simulink model "chaotic_controller_gt"  (R2025b)
settings: Solver=FixedStepDiscrete  StartTime=0.0  StopTime=300.0  FixedStep=0.1  RelTol=1e-3
settings Model: Creator=soumya2049  LastModifiedBy=aniket

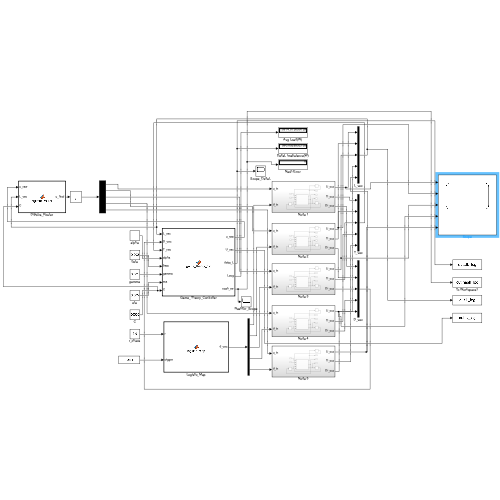
[thumbnail: Simulink's stored preview of the top-level diagram]
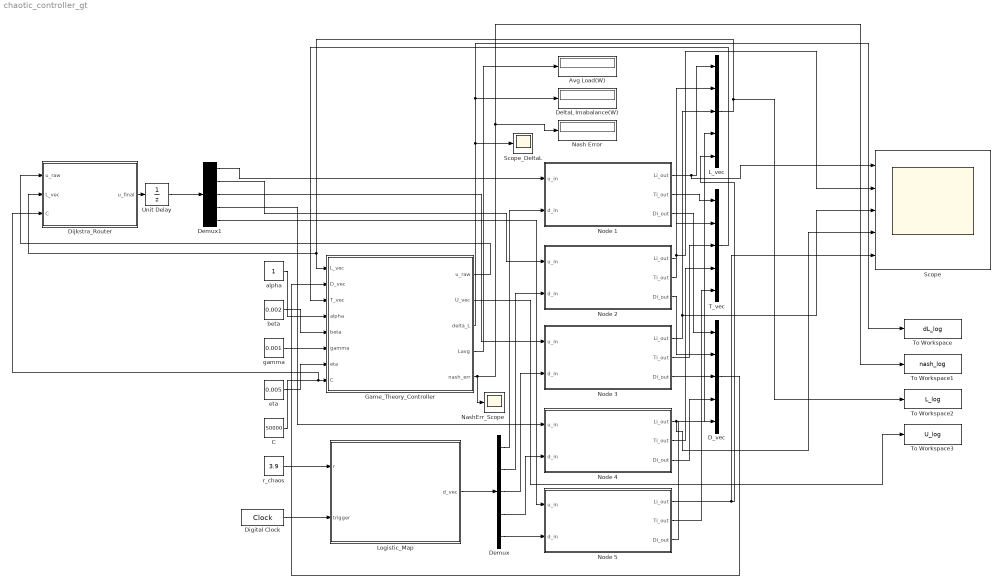
== system chaotic_controller_gt ==
  Avg Load(W) : Display
  C : Constant  Value=50000
  D_vec : Mux  Inputs=5
  DeltaL Imabalance(W) : Display
  Demux : Demux  Outputs=5
  Demux1 : Demux  Outputs=5
  Digital Clock : DigitalClock
  Dijkstra_Router : MATLAB Function  TreatAsAtomicUnit=on
  Game_Theory_Controller : MATLAB Function  TreatAsAtomicUnit=on
  L_vec : Mux  Inputs=5
  Logistic_Map : MATLAB Function  TreatAsAtomicUnit=on
  Nash Error : Display
  NashErr_Scope : Scope
  Node 1 : Subsystem
  Node 2 : Subsystem
  Node 3 : Subsystem
  Node 4 : Subsystem
  Node 5 : Subsystem
  Scope : Scope  NumInputPorts=5
      settings: ActiveDisplayYMinimum=-1436.8341921945957  ActiveDisplayYMaximum=13231.507729751364  DataLoggingVariableName=ScopeData2
  Scope_DeltaL : Scope
      settings: ActiveDisplayYMinimum=-1  ActiveDisplayYMaximum=1
  T_vec : Mux  Inputs=5
  To Workspace : ToWorkspace  VariableName=dL_log  SampleTime=-1
  To Workspace1 : ToWorkspace  VariableName=nash_log  SampleTime=-1
  To Workspace2 : ToWorkspace  VariableName=L_log  SampleTime=-1
  To Workspace3 : ToWorkspace  VariableName=U_log  SampleTime=-1
  Unit Delay : UnitDelay  InitialCondition=zeros(5,1)  SampleTime=-1  HasFrameUpgradeWarning=on
  alpha : Constant
  beta : Constant  Value=0.002
  eta : Constant  Value=0.005
  gamma : Constant  Value=0.001
  r_chaos : Constant  Value=3.9
  wires:
  Digital Clock/1 -> Logistic_Map/2(trigger)
  alpha/1 -> Game_Theory_Controller/4(alpha)
  Node 2/2(Ti_out) -> Scope/2, T_vec/2
  C/1 -> Dijkstra_Router/3(C), Game_Theory_Controller/8(C)
  beta/1 -> Game_Theory_Controller/5(beta)
  gamma/1 -> Game_Theory_Controller/6(gamma)
  r_chaos/1 -> Logistic_Map/1(r)
  Node 3/3(Di_out) -> D_vec/3
  eta/1 -> Game_Theory_Controller/7(eta)
  Logistic_Map/1(d_vec) -> Demux/1
  Demux/1 -> Node 1/2(d_in)
  Node 5/1(Li_out) -> Scope/5, L_vec/5
  Demux/2 -> Node 2/2(d_in)
  Demux/3 -> Node 3/2(d_in)
  Demux/4 -> Node 4/2(d_in)
  Demux/5 -> Node 5/2(d_in)
  Node 1/1(Li_out) -> Scope/1, L_vec/1
  Node 1/2(Ti_out) -> T_vec/1
  Node 5/3(Di_out) -> D_vec/5
  Node 1/3(Di_out) -> D_vec/1
  Node 2/1(Li_out) -> L_vec/2
  Node 2/3(Di_out) -> D_vec/2
  Node 3/1(Li_out) -> Scope/3, L_vec/3
  Node 3/2(Ti_out) -> T_vec/3
  Node 4/1(Li_out) -> Scope/4, L_vec/4
  Node 4/2(Ti_out) -> T_vec/4
  Node 4/3(Di_out) -> D_vec/4
  Node 5/2(Ti_out) -> T_vec/5
  L_vec/1 -> To Workspace2/1, Game_Theory_Controller/1(L_vec), Dijkstra_Router/2(L_vec)
  T_vec/1 -> Game_Theory_Controller/3(T_vec)
  D_vec/1 -> Game_Theory_Controller/2(D_vec)
  Game_Theory_Controller/1(u_raw) -> Dijkstra_Router/1(u_raw)
  Demux1/2 -> Node 2/1(u_in)
  Demux1/3 -> Node 3/1(u_in)
  Demux1/4 -> Node 4/1(u_in)
  Demux1/5 -> Node 5/1(u_in)
  Dijkstra_Router/1(u_final) -> Unit Delay/1
  Unit Delay/1 -> Demux1/1
  Game_Theory_Controller/3(delta_L) -> DeltaL Imabalance(W)/1, To Workspace/1, Scope_DeltaL/1
  Game_Theory_Controller/5(nash_err) -> Nash Error/1, To Workspace1/1, NashErr_Scope/1
  Game_Theory_Controller/2(U_vec) -> To Workspace3/1
  Game_Theory_Controller/4(Lavg) -> Avg Load(W)/1
  Demux1/1 -> Node 1/1(u_in)

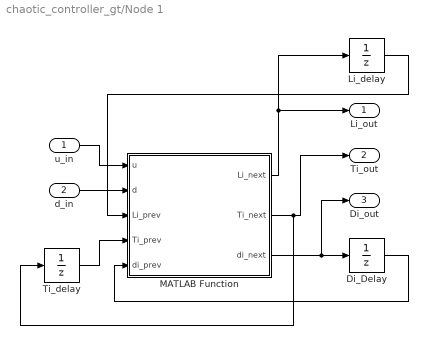
== system chaotic_controller_gt/Node 1 ==
  u_in : Inport
  d_in : Inport  Port=2
  Di_Delay : UnitDelay  InitialCondition=5000  SampleTime=-1  HasFrameUpgradeWarning=on
  Li_delay : UnitDelay  InitialCondition=3000  SampleTime=-1  HasFrameUpgradeWarning=on
  MATLAB Function : MATLAB Function  TreatAsAtomicUnit=on
  Ti_delay : UnitDelay  InitialCondition=30  SampleTime=-1  HasFrameUpgradeWarning=on
  Li_out : Outport
  Ti_out : Outport  Port=2
  Di_out : Outport  Port=3
  wires:
  MATLAB Function/2(Ti_next) -> Ti_delay/1, Ti_out/1
  u_in/1 -> MATLAB Function/1(u)
  d_in/1 -> MATLAB Function/2(d)
  Ti_delay/1 -> MATLAB Function/4(Ti_prev)
  MATLAB Function/1(Li_next) -> Li_out/1, Li_delay/1
  Di_Delay/1 -> MATLAB Function/5(di_prev)
  MATLAB Function/3(di_next) -> Di_out/1, Di_Delay/1
  Li_delay/1 -> MATLAB Function/3(Li_prev)

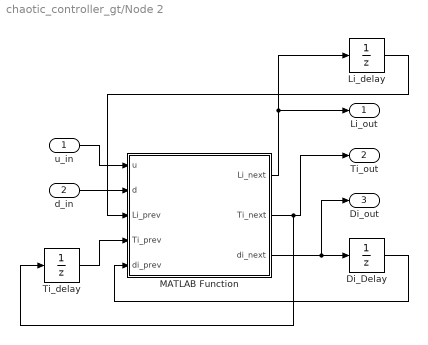
== system chaotic_controller_gt/Node 2 ==
  u_in : Inport
  d_in : Inport  Port=2
  Di_Delay : UnitDelay  InitialCondition=5000  SampleTime=-1  HasFrameUpgradeWarning=on
  Li_delay : UnitDelay  InitialCondition=3000  SampleTime=-1  HasFrameUpgradeWarning=on
  MATLAB Function : MATLAB Function  TreatAsAtomicUnit=on
  Ti_delay : UnitDelay  InitialCondition=30  SampleTime=-1  HasFrameUpgradeWarning=on
  Li_out : Outport
  Ti_out : Outport  Port=2
  Di_out : Outport  Port=3
  wires:
  MATLAB Function/2(Ti_next) -> Ti_delay/1, Ti_out/1
  u_in/1 -> MATLAB Function/1(u)
  d_in/1 -> MATLAB Function/2(d)
  Ti_delay/1 -> MATLAB Function/4(Ti_prev)
  MATLAB Function/1(Li_next) -> Li_out/1, Li_delay/1
  Di_Delay/1 -> MATLAB Function/5(di_prev)
  MATLAB Function/3(di_next) -> Di_out/1, Di_Delay/1
  Li_delay/1 -> MATLAB Function/3(Li_prev)

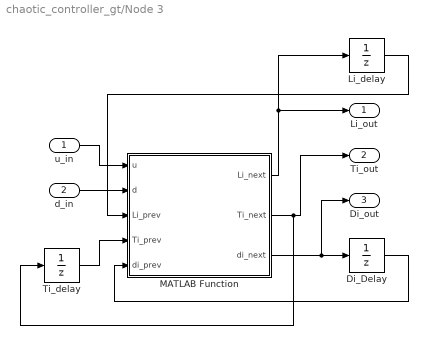
== system chaotic_controller_gt/Node 3 ==
  u_in : Inport
  d_in : Inport  Port=2
  Di_Delay : UnitDelay  InitialCondition=5000  SampleTime=-1  HasFrameUpgradeWarning=on
  Li_delay : UnitDelay  InitialCondition=3000  SampleTime=-1  HasFrameUpgradeWarning=on
  MATLAB Function : MATLAB Function  TreatAsAtomicUnit=on
  Ti_delay : UnitDelay  InitialCondition=30  SampleTime=-1  HasFrameUpgradeWarning=on
  Li_out : Outport
  Ti_out : Outport  Port=2
  Di_out : Outport  Port=3
  wires:
  MATLAB Function/2(Ti_next) -> Ti_delay/1, Ti_out/1
  u_in/1 -> MATLAB Function/1(u)
  d_in/1 -> MATLAB Function/2(d)
  Ti_delay/1 -> MATLAB Function/4(Ti_prev)
  MATLAB Function/1(Li_next) -> Li_out/1, Li_delay/1
  Di_Delay/1 -> MATLAB Function/5(di_prev)
  MATLAB Function/3(di_next) -> Di_out/1, Di_Delay/1
  Li_delay/1 -> MATLAB Function/3(Li_prev)

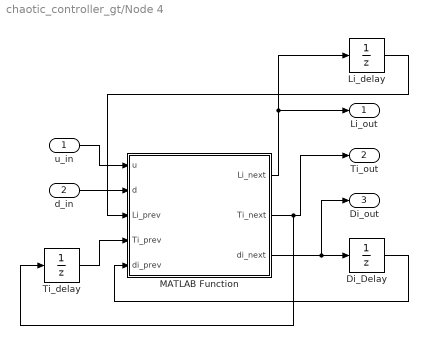
== system chaotic_controller_gt/Node 4 ==
  u_in : Inport
  d_in : Inport  Port=2
  Di_Delay : UnitDelay  InitialCondition=5000  SampleTime=-1  HasFrameUpgradeWarning=on
  Li_delay : UnitDelay  InitialCondition=3000  SampleTime=-1  HasFrameUpgradeWarning=on
  MATLAB Function : MATLAB Function  TreatAsAtomicUnit=on
  Ti_delay : UnitDelay  InitialCondition=30  SampleTime=-1  HasFrameUpgradeWarning=on
  Li_out : Outport
  Ti_out : Outport  Port=2
  Di_out : Outport  Port=3
  wires:
  MATLAB Function/2(Ti_next) -> Ti_delay/1, Ti_out/1
  u_in/1 -> MATLAB Function/1(u)
  d_in/1 -> MATLAB Function/2(d)
  Ti_delay/1 -> MATLAB Function/4(Ti_prev)
  MATLAB Function/1(Li_next) -> Li_out/1, Li_delay/1
  Di_Delay/1 -> MATLAB Function/5(di_prev)
  MATLAB Function/3(di_next) -> Di_out/1, Di_Delay/1
  Li_delay/1 -> MATLAB Function/3(Li_prev)

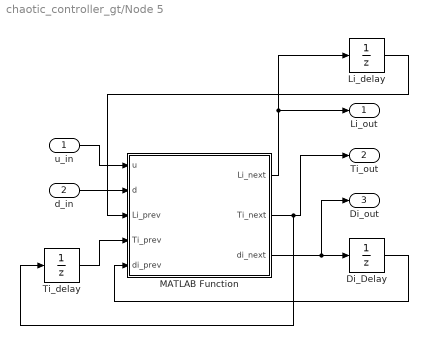
== system chaotic_controller_gt/Node 5 ==
  u_in : Inport
  d_in : Inport  Port=2
  Di_Delay : UnitDelay  InitialCondition=5000  SampleTime=-1  HasFrameUpgradeWarning=on
  Li_delay : UnitDelay  InitialCondition=3000  SampleTime=-1  HasFrameUpgradeWarning=on
  MATLAB Function : MATLAB Function  TreatAsAtomicUnit=on
  Ti_delay : UnitDelay  InitialCondition=30  SampleTime=-1  HasFrameUpgradeWarning=on
  Li_out : Outport
  Ti_out : Outport  Port=2
  Di_out : Outport  Port=3
  wires:
  MATLAB Function/2(Ti_next) -> Ti_delay/1, Ti_out/1
  u_in/1 -> MATLAB Function/1(u)
  d_in/1 -> MATLAB Function/2(d)
  Ti_delay/1 -> MATLAB Function/4(Ti_prev)
  MATLAB Function/1(Li_next) -> Li_out/1, Li_delay/1
  Di_Delay/1 -> MATLAB Function/5(di_prev)
  MATLAB Function/3(di_next) -> Di_out/1, Di_Delay/1
  Li_delay/1 -> MATLAB Function/3(Li_prev)

== matlab function chaotic_controller_gt/Dijkstra_Router ==
  data: u_raw input; u_final output; L_vec input; C input
function u_final = dijkstra_router(u_raw, L_vec, C)
%  u_raw  = 5×1 allocations from game theory (W)
%  L_vec  = 5×1 current loads (W) — used as edge weights
%  C      = capacity limit (W)
%  u_final = 5×1 optimally routed allocations (W)
%
%  DIJKSTRA INTERPRETATION:
%  Nodes = charging stations. Edge weight = current load.
%  "Shortest path" = lowest-load path for power delivery.
%  Heavily loaded nodes get throttled; underloaded get boosted.

total = sum(u_raw);

if total <= C
    u_final = u_raw;   % no congestion — pass through unchanged
    return;
end

%── Model 5 nodes as a weighted graph ─────────────────────────
%  Build a simple adjacency: nodes connected to a central bus
%  Edge weight = current load (W) — high load = costly path
Lavg      = mean(L_vec);
weights   = L_vec / max(L_vec);          % normalise (0 to 1)
distances = weights;                     % Dijkstra "distance" = load weight

%── Sort by Dijkstra distance (lowest load = shortest path) ───
[~, path_order] = sort(distances, 'ascend');  % underloaded nodes get priority

%── Distribute capacity along the optimal path ────────────────
scale   = C / total;
u_final = u_raw * scale;                    % base scaling

%── Redistribute along optimal path: boost underloaded nodes ──
saved = 0;
for k = 5:-1:3                               % top 3 highest-load nodes
    idx           = path_order(k);
    cut           = u_final(idx) * 0.15;      % take 15% from overloaded
    u_final(idx) = u_final(idx) - cut;
    saved         = saved + cut;
end
for k = 1:2                                  % give saved power to 2 underloaded
    idx           = path_order(k);
    u_final(idx) = u_final(idx) + saved/2;
end

%── Safety clamp ──────────────────────────────────────────────
u_final = max(0, min(u_final, 15000));
end

== matlab function chaotic_controller_gt/Node 2/MATLAB Function ==
  data: u input double; Li_next output double; d input double; Li_prev input double; Ti_prev input double; di_prev input double; Ti_next output double; di_next output double
function [Li_next, Ti_next, di_next] = node_dynamics(u, d, Li_prev, Ti_prev, di_prev)
%  u       = allocated power (W) — comes from Dijkstra router
%  d       = chaos disturbance (0 to 1) — from logistic map
%  Li_prev = load at previous timestep (W)
%  Ti_prev = temperature at previous timestep (°C)
%  di_prev = this node's strategy/demand at previous timestep (W)

%  Physical constants
dt    = 0.1;    % sample time (s)
beta  = 0.85;  % charging efficiency (fraction)
alpha = 0.04;  % thermal rise rate (°C per W·s)
eta_t = 0.002; % thermal dissipation coefficient
T_amb = 30;    % ambient temperature (°C)

%  Load update: current draws from allocation, disturbance adds noise
Li_next = Li_prev + dt * (u - beta * Li_prev) + d * 800;

%  Temperature update: rises with power, dissipates toward ambient
Ti_next = Ti_prev + dt * (alpha * u - eta_t * (Ti_prev - T_amb));

%  Strategy: node updates its demand toward allocated value
di_next = di_prev * 0.9 + u * 0.1;  % smoothed demand tracking

%  Hard physical limits
Li_next = max(0, min(Li_next, 15000));   % 0–15 kW
Ti_next = max(20, min(Ti_next, 65));     % 20–65°C
di_next = max(0, min(di_next, 15000));   % 0–15 kW
end

== matlab function chaotic_controller_gt/Node 1/MATLAB Function ==
  data: u input double; Li_next output double; d input double; Li_prev input double; Ti_prev input double; di_prev input double; Ti_next output double; di_next output double
function [Li_next, Ti_next, di_next] = node_dynamics(u, d, Li_prev, Ti_prev, di_prev)
%  u       = allocated power (W) — comes from Dijkstra router
%  d       = chaos disturbance (0 to 1) — from logistic map
%  Li_prev = load at previous timestep (W)
%  Ti_prev = temperature at previous timestep (°C)
%  di_prev = this node's strategy/demand at previous timestep (W)

%  Physical constants
dt    = 0.1;    % sample time (s)
beta  = 0.85;  % charging efficiency (fraction)
alpha = 0.04;  % thermal rise rate (°C per W·s)
eta_t = 0.002; % thermal dissipation coefficient
T_amb = 30;    % ambient temperature (°C)

%  Load update: current draws from allocation, disturbance adds noise
Li_next = Li_prev + dt * (u - beta * Li_prev) + d * 800;

%  Temperature update: rises with power, dissipates toward ambient
Ti_next = Ti_prev + dt * (alpha * u - eta_t * (Ti_prev - T_amb));

%  Strategy: node updates its demand toward allocated value
di_next = di_prev * 0.9 + u * 0.1;  % smoothed demand tracking

%  Hard physical limits
Li_next = max(0, min(Li_next, 15000));   % 0–15 kW
Ti_next = max(20, min(Ti_next, 65));     % 20–65°C
di_next = max(0, min(di_next, 15000));   % 0–15 kW
end

== matlab function chaotic_controller_gt/Node 3/MATLAB Function ==
  data: u input double; Li_next output double; d input double; Li_prev input double; Ti_prev input double; di_prev input double; Ti_next output double; di_next output double
function [Li_next, Ti_next, di_next] = node_dynamics(u, d, Li_prev, Ti_prev, di_prev)
%  u       = allocated power (W) — comes from Dijkstra router
%  d       = chaos disturbance (0 to 1) — from logistic map
%  Li_prev = load at previous timestep (W)
%  Ti_prev = temperature at previous timestep (°C)
%  di_prev = this node's strategy/demand at previous timestep (W)

%  Physical constants
dt    = 0.1;    % sample time (s)
beta  = 0.85;  % charging efficiency (fraction)
alpha = 0.04;  % thermal rise rate (°C per W·s)
eta_t = 0.002; % thermal dissipation coefficient
T_amb = 30;    % ambient temperature (°C)

%  Load update: current draws from allocation, disturbance adds noise
Li_next = Li_prev + dt * (u - beta * Li_prev) + d * 800;

%  Temperature update: rises with power, dissipates toward ambient
Ti_next = Ti_prev + dt * (alpha * u - eta_t * (Ti_prev - T_amb));

%  Strategy: node updates its demand toward allocated value
di_next = di_prev * 0.9 + u * 0.1;  % smoothed demand tracking

%  Hard physical limits
Li_next = max(0, min(Li_next, 15000));   % 0–15 kW
Ti_next = max(20, min(Ti_next, 65));     % 20–65°C
di_next = max(0, min(di_next, 15000));   % 0–15 kW
end

== matlab function chaotic_controller_gt/Node 4/MATLAB Function ==
  data: u input double; Li_next output double; d input double; Li_prev input double; Ti_prev input double; di_prev input double; Ti_next output double; di_next output double
function [Li_next, Ti_next, di_next] = node_dynamics(u, d, Li_prev, Ti_prev, di_prev)
%  u       = allocated power (W) — comes from Dijkstra router
%  d       = chaos disturbance (0 to 1) — from logistic map
%  Li_prev = load at previous timestep (W)
%  Ti_prev = temperature at previous timestep (°C)
%  di_prev = this node's strategy/demand at previous timestep (W)

%  Physical constants
dt    = 0.1;    % sample time (s)
beta  = 0.85;  % charging efficiency (fraction)
alpha = 0.04;  % thermal rise rate (°C per W·s)
eta_t = 0.002; % thermal dissipation coefficient
T_amb = 30;    % ambient temperature (°C)

%  Load update: current draws from allocation, disturbance adds noise
Li_next = Li_prev + dt * (u - beta * Li_prev) + d * 800;

%  Temperature update: rises with power, dissipates toward ambient
Ti_next = Ti_prev + dt * (alpha * u - eta_t * (Ti_prev - T_amb));

%  Strategy: node updates its demand toward allocated value
di_next = di_prev * 0.9 + u * 0.1;  % smoothed demand tracking

%  Hard physical limits
Li_next = max(0, min(Li_next, 15000));   % 0–15 kW
Ti_next = max(20, min(Ti_next, 65));     % 20–65°C
di_next = max(0, min(di_next, 15000));   % 0–15 kW
end

== matlab function chaotic_controller_gt/Node 5/MATLAB Function ==
  data: u input double; Li_next output double; d input double; Li_prev input double; Ti_prev input double; di_prev input double; Ti_next output double; di_next output double
function [Li_next, Ti_next, di_next] = node_dynamics(u, d, Li_prev, Ti_prev, di_prev)
%  u       = allocated power (W) — comes from Dijkstra router
%  d       = chaos disturbance (0 to 1) — from logistic map
%  Li_prev = load at previous timestep (W)
%  Ti_prev = temperature at previous timestep (°C)
%  di_prev = this node's strategy/demand at previous timestep (W)

%  Physical constants
dt    = 0.1;    % sample time (s)
beta  = 0.85;  % charging efficiency (fraction)
alpha = 0.04;  % thermal rise rate (°C per W·s)
eta_t = 0.002; % thermal dissipation coefficient
T_amb = 30;    % ambient temperature (°C)

%  Load update: current draws from allocation, disturbance adds noise
Li_next = Li_prev + dt * (u - beta * Li_prev) + d * 800;

%  Temperature update: rises with power, dissipates toward ambient
Ti_next = Ti_prev + dt * (alpha * u - eta_t * (Ti_prev - T_amb));

%  Strategy: node updates its demand toward allocated value
di_next = di_prev * 0.9 + u * 0.1;  % smoothed demand tracking

%  Hard physical limits
Li_next = max(0, min(Li_next, 15000));   % 0–15 kW
Ti_next = max(20, min(Ti_next, 65));     % 20–65°C
di_next = max(0, min(di_next, 15000));   % 0–15 kW
end

== matlab function chaotic_controller_gt/Logistic_Map ==
  data: r input; d_vec output; trigger input
function d_vec = logistic_map(r, trigger)
%  r       = chaos parameter. Use 3.9 for full chaos.
%  trigger = connect a Clock block here to update every timestep
%  d_vec   = 5×1 disturbance vector, all values in (0, 1)
%
%  The logistic map: X(n+1) = r * Xn * (1 - Xn)
%  At r = 3.9 this is fully chaotic — never repeats, bounded (0,1)

persistent xn;
if isempty(xn)
    rng(7);  % fixed seed → reproducible chaos for debugging
    xn = rand(5, 1) * 0.4 + 0.3;  % init away from 0 and 1 (unstable fixed points)
end

xn    = r .* xn .* (1 - xn);   % logistic update — all 5 nodes, different values
d_vec = xn;                      % output (0 to 1) — scale inside node block
end

== matlab function chaotic_controller_gt/Game_Theory_Controller ==
  data: L_vec input; u_raw output; D_vec input; T_vec input; alpha input; beta input; gamma input; eta input; C input; U_vec output; delta_L output; Lavg output; nash_err output
function [u_raw, U_vec, delta_L, Lavg, nash_err] = game_theory_ctrl(L_vec, D_vec, T_vec, alpha, beta, gamma, eta, C)
%─────────────────────────────────────────────────────────────────
%  INPUTS
%  L_vec  = 5×1 — current load at each node (W), measured
%  D_vec  = 5×1 — current demand/strategy of each node (W)
%  T_vec  = 5×1 — current temperature at each node (°C)
%  alpha  = reward weight (how much nodes want power)
%  beta   = overload penalty weight
%  gamma  = fairness/balancing weight
%  eta    = gradient ascent step size (learning rate)
%  C      = transformer/grid capacity limit (W)
%
%  OUTPUTS
%  u_raw    = 5×1 — new power allocation for each node (before Dijkstra)
%  U_vec    = 5×1 — payoff value for each node (for monitoring)
%  delta_L  = scalar — load imbalance (Lmax - Lmin), target: 0
%  Lavg     = scalar — average load across all nodes
%  nash_err = scalar — how far system is from Nash equilibrium
%─────────────────────────────────────────────────────────────────

N      = 5;                        % number of players/nodes
SumD   = sum(D_vec);              % total demand across all nodes
Lavg   = mean(L_vec);             % average load (broadcast to all)
delta_L = max(L_vec) - min(L_vec); % load imbalance (primary metric)

%── PAYOFF FUNCTION for each node ─────────────────────────────
%  U_i = α·d_i  −  β·[max(0, ΣD − C)]²/N  −  γ·(d_i − d_avg)²
overload    = max(0, SumD - C);               % excess beyond capacity
penalty_sys = beta * overload^2 / N;           % system-wide cost, shared equally
d_avg       = mean(D_vec);                      % average strategy
U_vec       = alpha .* D_vec - penalty_sys - gamma .* (D_vec - d_avg).^2;

%── GRADIENT ASCENT — each node updates its strategy ──────────
%  ∂U_i/∂d_i = α − (2β/N)·max(0,ΣD−C) − 2γ·(d_i − d_avg)
grad = alpha - (2*beta/N) .* overload - 2*gamma .* (D_vec - d_avg);

%── TEMPERATURE PENALTY — throttle hot nodes ──────────────────
%  Nodes above 45°C get their gradient reduced
temp_penalty = max(0, (T_vec - 45) ./ 20);    % 0 below 45°C, up to 1 at 65°C
grad         = grad .* (1 - temp_penalty);         % reduce ascent for hot nodes

%── NEW STRATEGY = old strategy + learning_rate × gradient ────
D_new = D_vec + eta .* grad;

%── CLAMP strategies to physical limits ───────────────────────
D_new = max(500, min(D_new, 15000));     % 500W min (keep node alive), 15kW max

%── NASH ERROR — measure distance from equilibrium ────────────
%  At Nash: all gradients ≈ 0. Nash error = norm of gradient vector.
nash_err = norm(grad);                       % target: approaches 0

%── ALLOCATE based on new strategies ─────────────────────────
%  u_raw goes to Dijkstra next for routing optimisation
u_raw = D_new;
end
